simulink model "base_model_lqeH"  (R2020b)
settings: Solver=ode1  StartTime=0  StopTime=1150  FixedStep=0.1  RelTol=1e-3
libraries: simulink_extras x33
(part 1 of 3)
settings Model: Creator=LEON  LastModifiedBy=leonk
settings DataIOCC: ReturnWorkspaceOutputs=off
settings OptimizationCC: DefaultParameterBehavior=Inlined  EnhancedBackFolding=on  PassReuseOutputArgsAs=Individual arguments  ZeroExternalMemoryAtStartup=off  ZeroInternalMemoryAtStartup=off  OptimizeBlockOrder=speed  DifferentSizesBufferReuse=on  OptimizationCustomize=off  EfficientTunableParamExpr=on
settings DebuggingCC: ParameterTunabilityLossMsg=error  ArithmeticOperatorsInVariantConditions=warning
settings SFSimCC: MATLABDynamicMemAlloc=off  CustomCodeUndefinedFunction=UseInterfaceOnly
settings RTWCC: Description=Embedded Coder  SystemTargetFile=ert.tlc  GenCodeOnly=on  TemplateMakefile=ert_default_tmf
settings CodeAppCC: ForceParamTrailComments=on  IgnoreCustomStorageClasses=off  OperatorAnnotations=on  SimulinkDataObjDesc=on  SFDataObjDesc=on  InsertBlockDesc=on
settings ERTTargetCC: TargetLangStandard=C99 (ISO)  GenerateSampleERTMain=on  InlinedParameterPlacement=NonHierarchical  ERTCustomFileTemplate=example_file_process.tlc

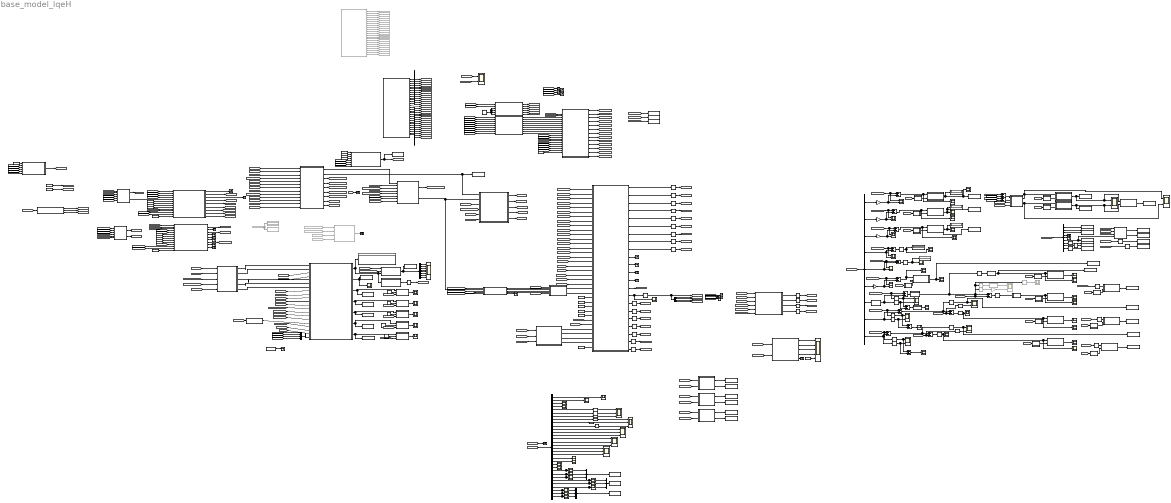
== system base_model_lqeH ==
  note: alpha&betta&gamma
  note: Ve&Vn
  note: lat&lon
  note: sat2Params
  note: sat3Params
  note: sat1Params
  note: time
  note: Altitude
  note: Алгориттм БИНС
  note: Егор
  note: Без базового спутника
  note: Корнтроль измерений
  note: Autoreloader
     {21..22,24,28..33,40..50} (20 alike) : Scope
     {23,26..27,34..35,37..39} (8 alike) : Scope  NumInputPorts=2
  "   25" : Scope  Commented=on  NumInputPorts=2
  "   36" : Scope  Commented=on
  "  3" : Scope
  " 12" : Scope
  " 13" : Scope
  " 14" : Scope  NumInputPorts=2
  " 15" : Scope  NumInputPorts=2
  " 16" : Scope  NumInputPorts=2
  ADD error SAT : MATLAB Function  TreatAsAtomicUnit=on
  Constant{,3..5,8..14,34,36} (13 alike) : Constant  Value=0
  Constant1 : Constant
  Constant{15,19..20,22} (4 alike) : Constant  OutDataTypeStr=uint8
  Constant16 : Constant  Value=[1, 1, 0.4, 10]
  Constant17 : Constant  Value=3
  Constant18 : Constant  Value=8  OutDataTypeStr=uint8
  Constant2 : Constant  Value=15
  Constant21 : Constant  Value=0  OutDataTypeStr=uint8
  Constant23 : Constant  Value=1000
  Constant28 : Constant  Value=8
  Constant29 : Constant  Value=50
  Constant30 : Constant  Value=0  OutDataTypeStr=uint8
  Constant31 : Constant  Value=500
  Constant32 : Constant  Value=800
  Constant33 : Constant  Value=1200
  Constant35 : Constant
  Constant6 : Constant  Value=10
  Constant7 : Constant  Value=10
  DOPS : MATLAB Function  TreatAsAtomicUnit=on
  Demux : Demux  Outputs=32
  Demux2 : Demux
  Demux4 : Demux  Outputs=8
  Demux5 : Demux  Outputs=9
  Demux6 : Demux  Outputs=9
  Display11 : Display  Commented=on
  Display{12,23,29..32} (6 alike) : Display
  FormZ : MATLAB Function  TreatAsAtomicUnit=on
  From168 : From  Commented=on  GotoTag=satVisible
  From270 : From  Commented=on  GotoTag=psdRange_GNSSvis
  From289 : From  Commented=on  GotoTag=satCoefs
  From291 : From  Commented=on  GotoTag=satIDvis
  From298 : From  Commented=on  GotoTag=satInctrl
  Fuck matlab1 : MATLAB Function  TreatAsAtomicUnit=on
  Fuck matlab10 : MATLAB Function  Commented=on  TreatAsAtomicUnit=on
  Fuck matlab11 : MATLAB Function  TreatAsAtomicUnit=on
  Fuck matlab2 : MATLAB Function  TreatAsAtomicUnit=on
  Fuck matlab3 : MATLAB Function  TreatAsAtomicUnit=on
  Fuck matlab4 : MATLAB Function  TreatAsAtomicUnit=on
  Fuck matlab5 : MATLAB Function  TreatAsAtomicUnit=on
  Fuck matlab6 : MATLAB Function  TreatAsAtomicUnit=on
  Fuck matlab7 : MATLAB Function  TreatAsAtomicUnit=on
  Fuck matlab8 : MATLAB Function  TreatAsAtomicUnit=on
  Fuck matlab9 : MATLAB Function  TreatAsAtomicUnit=on
  GNNS_freq_imitetor : MATLAB Function  TreatAsAtomicUnit=on
  GNNS_freq_imitetor1 : MATLAB Function  TreatAsAtomicUnit=on
  GNSS_integrity_control1 : MATLAB Function  TreatAsAtomicUnit=on
  GNSS_receiver_imitator10 : MATLAB Function  TreatAsAtomicUnit=on
  GNSS_receiver_imitator6 : MATLAB Function  TreatAsAtomicUnit=on
  GNSS_receiver_imitator7 : MATLAB Function  TreatAsAtomicUnit=on
  GNSS_receiver_imitator8 : MATLAB Function  TreatAsAtomicUnit=on
  GNSS_receiver_imitator9 : MATLAB Function  TreatAsAtomicUnit=on
  GSK->DGSK : MATLAB Function  TreatAsAtomicUnit=on
  GSK->DGSK1 : MATLAB Function  TreatAsAtomicUnit=on
  Goto1 : Goto  Commented=on  GotoTag=ACC_data
  Goto10 : Goto  Commented=on  GotoTag=ic_Vh
  Goto11 : Goto  Commented=on  GotoTag=time_shift
  Goto112 : Goto  Commented=on  GotoTag=satStartTime
  Goto12 : Goto  Commented=on  GotoTag=GRS_data
  Goto129 : Goto  Commented=on  GotoTag=offSet_Vn
  Goto136 : Goto  Commented=on  GotoTag=satStopTime
  Goto137 : Goto  Commented=on  GotoTag=offSet_Ve
  Goto138 : Goto  Commented=on  GotoTag=offSet_Vh
  Goto139 : Goto  Commented=on  GotoTag=offSet_lat
  Goto140 : Goto  Commented=on  GotoTag=offSet_lon
  Goto141 : Goto  Commented=on  GotoTag=offSet_alt
  Goto145 : Goto  Commented=on  GotoTag=satDeltaUp
  Goto146 : Goto  Commented=on  GotoTag=satDeltaDown
  Goto2 : Goto  Commented=on  GotoTag=ic_heading
  Goto3 : Goto  Commented=on  GotoTag=ic_pitch
  Goto4 : Goto  Commented=on  GotoTag=ic_roll
  Goto48 : Goto  Commented=on  GotoTag=ctrl_data
  Goto5 : Goto  Commented=on  GotoTag=ic_lat
  Goto6 : Goto  Commented=on  GotoTag=ic_lon
  Goto7 : Goto  Commented=on  GotoTag=ic_Ve
  Goto8 : Goto  Commented=on  GotoTag=ic_Vn
  Goto9 : Goto  Commented=on  GotoTag=ic_alt
  INS mesurment model : MATLAB Function  TreatAsAtomicUnit=on
  MATLAB Function3 : MATLAB Function  Commented=on  TreatAsAtomicUnit=on
  MATLAB Function4 : MATLAB Function  TreatAsAtomicUnit=on
  Memory{1,16..27,29..37} (22 alike) : Memory
  Model : ModelReference  ModelNameDialog=SINS_model_3ch_h.slx  SimulationMode=Normal  ModelReferenceVersion=5.358
  Model2 : ModelReference  ModelNameDialog=lqe_ins_h.slx  SimulationMode=Normal  ModelReferenceVersion=5.1159
  Mux : Mux  Inputs=3
  Mux1 : Mux  Inputs=3
  Mux2 : Mux  Inputs=3
  Mux3 : Mux
  Pitch_1 : simulink_extras/Transformations/Radians to Degrees
  Pitch_err   1 : simulink_extras/Transformations/Radians to Degrees
  Radians to Degrees{,13..14,17..19,22,27..29,31} (11 alike) : simulink_extras/Transformations/Radians to Degrees
  Radians to Degrees21 : simulink_extras/Transformations/Radians to Degrees  Commented=on
  Roll_err   1 : simulink_extras/Transformations/Radians to Degrees
  Scope{1..2,5..7,10..11,13..14,20..22,24..25,66,76..84} (24 alike) : Scope
  Scope{19,32,56..58} (5 alike) : Scope  NumInputPorts=3
  Scope3 : Scope  NumInputPorts=2
  Scope64 : Scope  NumInputPorts=8
  Scope8 : Scope  NumInputPorts=2
  Scope87 : Scope  NumInputPorts=5
  Scope9 : Scope  NumInputPorts=2
  StaPosition : MATLAB Function  TreatAsAtomicUnit=on
  Terminator{,1..27} (28 alike) : Terminator
  To Workspace1 : ToWorkspace  Commented=on  VariableName=satVisibleCount  SampleTime=-1
  To Workspace10 : ToWorkspace  VariableName=satIC_2cfs  SampleTime=-1
  To Workspace11 : ToWorkspace  VariableName=satIC_3cfs  SampleTime=-1
  To Workspace12 : ToWorkspace  VariableName=satIC_3ID  SampleTime=-1
  To Workspace13 : ToWorkspace  VariableName=satIC_1P  SampleTime=-1
  To Workspace14 : ToWorkspace  VariableName=satIC_2P  SampleTime=-1
  To Workspace15 : ToWorkspace  VariableName=d_heading  SampleTime=-1
  To Workspace16 : ToWorkspace  VariableName=satIC_3P  SampleTime=-1
  To Workspace17 : ToWorkspace  VariableName=pitch_err  SampleTime=-1
  To Workspace18 : ToWorkspace  VariableName=roll_err  SampleTime=-1
  To Workspace19 : ToWorkspace  VariableName=d_roll  SampleTime=-1
  To Workspace2 : ToWorkspace  VariableName=slowZLevel  SampleTime=-1
  To Workspace20 : ToWorkspace  VariableName=Ve_REF  SampleTime=-1
  To Workspace21 : ToWorkspace  VariableName=Vn_REF  SampleTime=-1
  To Workspace22 : ToWorkspace  VariableName=Vh_REF  SampleTime=-1
  To Workspace23 : ToWorkspace  VariableName=Y_REF  SampleTime=-1
  To Workspace24 : ToWorkspace  VariableName=X_REF  SampleTime=-1
  To Workspace25 : ToWorkspace  VariableName=alt_REF  SampleTime=-1
  To Workspace26 : ToWorkspace  VariableName=heading_REF  SampleTime=-1
  To Workspace27 : ToWorkspace  VariableName=pitch_REF  SampleTime=-1
  To Workspace28 : ToWorkspace  VariableName=roll_REF  SampleTime=-1
  To Workspace29 : ToWorkspace  VariableName=lat_REF  SampleTime=-1
  To Workspace3 : ToWorkspace  VariableName=latSINS  SampleTime=-1
  To Workspace30 : ToWorkspace  VariableName=lon_REF  SampleTime=-1
  To Workspace31 : ToWorkspace  VariableName=Ve_err  SampleTime=-1
  To Workspace32 : ToWorkspace  VariableName=Vn_err  SampleTime=-1
  To Workspace33 : ToWorkspace  VariableName=Vh_err  SampleTime=-1
  To Workspace34 : ToWorkspace  VariableName=lat_err  SampleTime=-1
  To Workspace35 : ToWorkspace  VariableName=lon_err  SampleTime=-1
  To Workspace36 : ToWorkspace  VariableName=alt_err  SampleTime=-1
  To Workspace37 : ToWorkspace  VariableName=heading_err  SampleTime=-1
  To Workspace38 : ToWorkspace  VariableName=intCtrl_status  SampleTime=-1
  To Workspace39 : ToWorkspace  VariableName=fastCriteriaLevel  SampleTime=-1
  To Workspace4 : ToWorkspace  VariableName=psdErr  SampleTime=-1
  To Workspace40 : ToWorkspace  VariableName=slowMeanLevel  SampleTime=-1
  To Workspace41 : ToWorkspace  VariableName=fastLevel  SampleTime=-1
  To Workspace42 : ToWorkspace  VariableName=lonSINS  SampleTime=-1
  To Workspace43 : ToWorkspace  VariableName=altSINS  SampleTime=-1
  To Workspace44 : ToWorkspace  VariableName=slowZCriteria  SampleTime=-1
  To Workspace45 : ToWorkspace  VariableName=satVisibleCount  SampleTime=-1
  To Workspace46 : ToWorkspace  VariableName=crdErr  SampleTime=-1
  To Workspace5 : ToWorkspace  VariableName=satAV  SampleTime=-1
  To Workspace6 : ToWorkspace  VariableName=d_pitch  SampleTime=-1
  To Workspace7 : ToWorkspace  VariableName=satIC_1ID  SampleTime=-1
  To Workspace8 : ToWorkspace  VariableName=satIC_1cfs  SampleTime=-1
  To Workspace9 : ToWorkspace  VariableName=satIC_2ID  SampleTime=-1
  "Ve_err   " : Sum  Inputs=+-
  Ve_err 1 : MATLAB Function  TreatAsAtomicUnit=on
  "Vh_err  " : Sum  Inputs=+-
  Vh_err 1 : MATLAB Function  TreatAsAtomicUnit=on
  "Vn_err  " : Sum  Inputs=+-
  Vn_err 1 : MATLAB Function  TreatAsAtomicUnit=on
  "alt_err    " : Sum  Inputs=+-
  alt_err 1 : MATLAB Function  TreatAsAtomicUnit=on
  altimetrImitator : MATLAB Function  TreatAsAtomicUnit=on
  altimetrImitator1 : MATLAB Function  TreatAsAtomicUnit=on
  bigHeadingFix1 : MATLAB Function  TreatAsAtomicUnit=on
  bigHeadingFix2 : MATLAB Function  TreatAsAtomicUnit=on
  coord_err7 : MATLAB Function  TreatAsAtomicUnit=on
  coord_err8 : MATLAB Function  TreatAsAtomicUnit=on
  crtl_Ve1 : Gain
  crtl_Vh1 : Gain
  crtl_Vn1 : Gain
  crtl_altitude1 : Gain
  d_heading1 : Gain  Commented=on
  d_pitch1 : simulink_extras/Transformations/Radians to Degrees
  d_roll1 : simulink_extras/Transformations/Radians to Degrees
  heading_3 : simulink_extras/Transformations/Radians to Degrees
  heading_4 : simulink_extras/Transformations/Radians to Degrees  Commented=on
  heading_5 : simulink_extras/Transformations/Radians to Degrees  Commented=on
  heading_6 : simulink_extras/Transformations/Radians to Degrees
  heading_INS  1 : MATLAB Function  Commented=on  TreatAsAtomicUnit=on
  heading_INS  2 : MATLAB Function  TreatAsAtomicUnit=on
  "heading_err     " : MATLAB Function  TreatAsAtomicUnit=on
  heading_err     1 : MATLAB Function  TreatAsAtomicUnit=on
  heading_err     2 : MATLAB Function  TreatAsAtomicUnit=on
  heading_err     3 : MATLAB Function  TreatAsAtomicUnit=on
  heading_err     4 : MATLAB Function  TreatAsAtomicUnit=on
  heading_err    {1..9} (9 alike) : simulink_extras/Transformations/Radians to Degrees
  heading_err  1 : MATLAB Function  TreatAsAtomicUnit=on
  heading_err1 : Sum  Inputs=+-
  heading_err_FBon 2 : MATLAB Function  TreatAsAtomicUnit=on
  heading_err_FBon1 : Sum  Inputs=+-
  lat_err 1 : MATLAB Function  TreatAsAtomicUnit=on
  lat_err 2 : MATLAB Function  TreatAsAtomicUnit=on
  lat_err3 : Sum  Inputs=+-
  lat_err4 : Sum  Inputs=+-
  lon_err 1 : MATLAB Function  TreatAsAtomicUnit=on
  lon_err3 : Sum  Inputs=+-
  lon_err4 : Sum  Inputs=+-
  lqe_coord_cor2 : MATLAB Function  TreatAsAtomicUnit=on
  "pitch_err    " : MATLAB Function  TreatAsAtomicUnit=on
  pitch_err 1 : simulink_extras/Transformations/Radians to Degrees
  pitch_err1 : Sum  Inputs=+-
  pitch_err_FBon1 : Sum  Inputs=+-
  psdRange_Sat : ModelReference  ModelNameDialog=psdRange_model.slx  SimulationMode=Normal  ModelReferenceVersion=1.113
      settings: PortSchema="{\"entries\":[{\"content\":{\"sides\":[{\"content\":{\"connectorIds\":[\"In1\",\"In2\",\"In3\",\"In4\",\"In5\",\"In6\",\"In8\",\"In7\",\"In9\",\"In10\",\"In11\",\"In12\",\"In13\",\"In14\"]},\"type\":\"ConnectorPlacement.EquallySpacedRectSide\",\"uuid\":\"0992fbca-6c1d-43ca-af68-52a1663360d0\"},{\"content\":{\"connectorIds\":[\"Out1\",\"Out2\",\"Out3\",\"Out4\",\"Out5\",\"Out6\",\"Out7\",\"Out8\",\"Out9\"],\"side\":\"RIGHT\"},\"type\":\"ConnectorPlacement.EquallySpacedRectSide\",\"uuid\":\"279fbf8e-dc69-40a1-ad66-d0ae37456352\"},{\"content\":{\"connectorIds\":[],\"side\":\"TOP\"},\"type\":\"ConnectorPlacement.EquallySpacedRectSide\",\"uuid\":\"4e5886c2-56d5-49fe-96a3-fea858babac4\"},{\"content\":{\"connectorIds\":[],\"side\":\"HIDDEN\"},\"type\":\"ConnectorPlacement.EquallySpacedRectSide\",\"uuid\":\"b5bcda28-ff0f-4448-99fe-4545b2b7e269\"}]},\"type\":\"ConnectorPlacement.EquallySpacedConnector\",\"uuid\":\"877d5e3f-f6cf-4aa5-86c3-e38699d2b886\"}],\"packageUris\":[\"http://schema.mathworks.com/mf0/Connector/R2020b\"],\"version\":\"1.0\"}"
  psdRange_Sat1 : ModelReference  ModelNameDialog=psdRange_model.slx  SimulationMode=Normal  ModelReferenceVersion=1.113
      settings: PortSchema="{\"entries\":[{\"content\":{\"sides\":[{\"content\":{\"connectorIds\":[\"In1\",\"In2\",\"In3\",\"In4\",\"In5\",\"In6\",\"In8\",\"In7\",\"In9\",\"In10\",\"In11\",\"In12\",\"In13\",\"In14\"]},\"type\":\"ConnectorPlacement.EquallySpacedRectSide\",\"uuid\":\"0992fbca-6c1d-43ca-af68-52a1663360d0\"},{\"content\":{\"connectorIds\":[\"Out1\",\"Out2\",\"Out3\",\"Out4\",\"Out5\",\"Out6\",\"Out7\",\"Out8\",\"Out9\"],\"side\":\"RIGHT\"},\"type\":\"ConnectorPlacement.EquallySpacedRectSide\",\"uuid\":\"279fbf8e-dc69-40a1-ad66-d0ae37456352\"},{\"content\":{\"connectorIds\":[],\"side\":\"TOP\"},\"type\":\"ConnectorPlacement.EquallySpacedRectSide\",\"uuid\":\"4e5886c2-56d5-49fe-96a3-fea858babac4\"},{\"content\":{\"connectorIds\":[],\"side\":\"HIDDEN\"},\"type\":\"ConnectorPlacement.EquallySpacedRectSide\",\"uuid\":\"b5bcda28-ff0f-4448-99fe-4545b2b7e269\"}]},\"type\":\"ConnectorPlacement.EquallySpacedConnector\",\"uuid\":\"877d5e3f-f6cf-4aa5-86c3-e38699d2b886\"}],\"packageUris\":[\"http://schema.mathworks.com/mf0/Connector/R2020b\"],\"version\":\"1.0\"}"
  roll_1 : simulink_extras/Transformations/Radians to Degrees
  "roll_err     " : MATLAB Function  TreatAsAtomicUnit=on
  roll_err 1 : simulink_extras/Transformations/Radians to Degrees
  roll_err{4..7} (4 alike) : Sum  Inputs=+-
  roll_err_FBon1 : Sum  Inputs=+-
  seter1 : MATLAB Function  TreatAsAtomicUnit=on
  seter10 : MATLAB Function  TreatAsAtomicUnit=on
  seter11 : MATLAB Function  TreatAsAtomicUnit=on
  seter12 : MATLAB Function  TreatAsAtomicUnit=on
  seter13 : MATLAB Function  TreatAsAtomicUnit=on
  seter2 : MATLAB Function  TreatAsAtomicUnit=on
  seter3 : MATLAB Function  TreatAsAtomicUnit=on
  seter4 : MATLAB Function  TreatAsAtomicUnit=on
  seter5 : MATLAB Function  TreatAsAtomicUnit=on
  seter6 : MATLAB Function  TreatAsAtomicUnit=on
  seter7 : MATLAB Function  TreatAsAtomicUnit=on
  seter8 : MATLAB Function  TreatAsAtomicUnit=on
  seter9 : MATLAB Function  TreatAsAtomicUnit=on
  wires:
  MATLAB Function3/1(GRS) -> Goto12/1
  MATLAB Function3/2(ACC) -> Goto1/1
  MATLAB Function3/3(heading) -> Goto2/1
  MATLAB Function3/4(pitch) -> Goto3/1
  MATLAB Function3/5(roll) -> Goto4/1
  MATLAB Function3/7(lon) -> Goto6/1
  MATLAB Function3/6(lat) -> Goto5/1
  MATLAB Function3/8(Ve) -> Goto7/1
  MATLAB Function3/9(Vn) -> Goto8/1
  MATLAB Function3/12(time_shft) -> Goto11/1
  MATLAB Function3/11(Vh) -> Goto10/1
  MATLAB Function3/10(H) -> Goto9/1
  Model/1 -> [SINS_Ve]
  Model/2 -> [SINS_Vn]
  Model/4 -> [SINS_latitude]
  Model/3 -> [SINS_Vh]
  Model/5 -> [SINS_longitude]
  Demux/14 -> Scope32/1
  Demux/4 -> Scope24/1
  Radians to Degrees13/1 -> Scope19/2
  Demux/15 -> Scope32/2
  Demux/7 -> Radians to Degrees14/1
  Radians to Degrees/1 -> Scope19/1
  Demux/16 -> Scope32/3
  Demux/5 -> Radians to Degrees/1
  Demux/6 -> Radians to Degrees13/1
  Demux/1 -> Scope20/1
  Demux/3 -> Scope22/1
  Radians to Degrees14/1 -> Scope19/3
  Demux/2 -> Scope21/1
  [GRS_data] -> INS mesurment model/1(grs_ideal)
  [ACC_data] -> INS mesurment model/2(acc_ideal)
  [ic_roll] -> lqe_coord_cor2/3(roll)
  [ic_pitch] -> lqe_coord_cor2/2(pitch)
  [ic_heading] -> lqe_coord_cor2/1(heading)
  [ic_Vn] -> lqe_coord_cor2/8(Vn)
  [ic_Ve] -> lqe_coord_cor2/7(Ve)
  [ic_lat] -> lqe_coord_cor2/4(lat)
  [ic_lon] -> lqe_coord_cor2/5(lon)
  Demux/8 -> Radians to Degrees17/1
  Demux/9 -> Radians to Degrees18/1
  Demux/10 -> Radians to Degrees19/1
  Demux/17 -> Scope58/1
  Demux/18 -> Scope58/2
  Demux/19 -> Scope58/3
  Radians to Degrees17/1 -> Scope56/1
  Demux/12 -> Scope57/2
  Demux/13 -> Scope57/3
  Demux/11 -> Scope57/1
  Radians to Degrees18/1 -> Scope56/2
  Radians to Degrees19/1 -> Scope56/3
  INS mesurment model/1(grs_data) -> [GRS_real]
  INS mesurment model/2(acc_data) -> [ACC_real]
  Model/7 -> [SINS_heading]
  Model/8 -> [SINS_pitch]
  Model/9 -> [SINS_roll]
  Model/10 -> [SINS_nGSK]
  Model/11 -> [SINS_OmgGSK]
  Model/12 -> [SINS_matDirCos]
  Model/6 -> [SINS_altitude]
  [amnd_matDirCos] -> Model/13
  Constant12/1 -> Model/21
  [ic_Vh] -> lqe_coord_cor2/9(Vh)
  [ic_alt] -> lqe_coord_cor2/6(alt)
  Demux/20 -> Scope76/1
  Demux/21 -> Scope5/1
  [time_shift] -> Model/20
  [lqe_dVn] -> Model/18
  [lqe_dVe] -> Model/17
  [lqe_dlon] -> Model/15
  [lqe_dlat] -> Model/14
  [lqe_dalt] -> Model/16
  [lqe_dVh] -> Model/19
  [lqe_ctrl] -> Model/12
  lqe_coord_cor2/9(Vh_0) -> Model/11
  lqe_coord_cor2/8(Vn_0) -> Model/10
  lqe_coord_cor2/7(Ve_0) -> Model/9
  lqe_coord_cor2/6(alt_0) -> Model/8
  lqe_coord_cor2/5(lon_0) -> Model/7
  lqe_coord_cor2/1(heading_0) -> Model/3
  lqe_coord_cor2/2(pitch_0) -> Model/4
  lqe_coord_cor2/3(roll_0) -> Model/5
  lqe_coord_cor2/4(lat_0) -> Model/6
  MATLAB Function3/13(cntrl_data) -> Goto48/1
  [ACC_real] -> Model/2
  [GRS_real] -> Model/1
  Model/13 -> [SINS_dVGSK]
  INS mesurment model/6(dK_grs) -> [dKgrs]
  Constant/1 -> INS mesurment model/4(n2), INS mesurment model/3(n1), INS mesurment model/5(n3), INS mesurment model/6(n4)
  INS mesurment model/3(dacc) -> [dacc]
  INS mesurment model/4(dgrs) -> [dgrs]
  INS mesurment model/5(dK_acc) -> [dKacc]
  [time_shift] -> StaPosition/1(time_shift)
  StaPosition/1(satCounter) -> [satCount]
  StaPosition/2(satPosVel) -> [satPosVel]
  Constant2/1 -> [elevMask]
  psdRange_Sat/1 -> Terminator/1
  psdRange_Sat/2 -> [psdRange_sat]
  psdRange_Sat/3 -> Terminator1/1
  psdRange_Sat/4 -> [psdVel_sat]
  StaPosition/3(satHealth) -> [satHealth]
  psdRange_Sat/5 -> [dPsdRange]
  [satVisible] -> FormZ/1(satVisible)
  [satCount] -> FormZ/2(satCount)
  psdRange_Sat/6 -> [satVisible]
  [satVisibleFlag_GNSS] -> FormZ/4(satVisibleFlag_GNSS)
  psdRange_Sat1/2 -> Terminator2/1
  psdRange_Sat1/4 -> Terminator3/1
  psdRange_Sat1/3 -> [psdVel_INS]
  psdRange_Sat1/1 -> [psdRange_INS]
  [psdVel_INS] -> FormZ/7(psdVel_INS)
  [psdRange_INS] -> FormZ/6(psdRange_INS)
  [psdRange_sat] -> FormZ/5(psdRange_sat)
  [psdVel_sat] -> FormZ/8(psdVel_sat)
  [time_shift] -> GNNS_freq_imitetor/3(time_shift)
  GNNS_freq_imitetor/1(satInfo) -> [satInfo_shrt]
  GNNS_freq_imitetor/3(timeDelay) -> [timeDelayGNSS]
  GNNS_freq_imitetor/4(frameAvalible_GNSS) -> [frameAvalible]
  psdRange_Sat1/5 -> Terminator4/1
  psdRange_Sat1/6 -> Terminator5/1
  FormZ/2(satNum) -> To Workspace45/1, GNNS_freq_imitetor/1(satNum_AV)
  GSK->DGSK1/1(pos) -> [posObjINS]
  GSK->DGSK1/2(vel) -> [velObjINS]
  FormZ/3(psdRange_INS_short) -> [psdRange_INSvis]
  FormZ/1(satInfo) -> ADD error SAT/1(satInfo)
  [GRS_real] -> Model2/11
  [SINS_dVGSK] -> Model2/15
  [ACC_real] -> Model2/13
  [SINS_nGSK] -> Model2/14
  [SINS_latitude] -> Model2/1
  [SINS_altitude] -> Model2/3
  [SINS_Vh] -> Model2/6
  [SINS_OmgGSK] -> Model2/12
  [SINS_roll] -> Model2/9
  [SINS_Vn] -> Model2/5
  [SINS_longitude] -> Model2/2
  [SINS_Ve] -> Model2/4
  [SINS_pitch] -> Model2/8
  [time_shift] -> Model2/16
  [SINS_matDirCos] -> Model2/10
  [SINS_heading] -> Model2/7
  Constant18/1 -> [satCountPreset]
  [satPosVel] -> psdRange_Sat/2
  [satHealth] -> psdRange_Sat/3
  [satCount] -> psdRange_Sat/1
  GSK->DGSK/2(vel) -> psdRange_Sat/5
  Constant8/1 -> psdRange_Sat/6
  Constant4/1 -> psdRange_Sat/7
  Constant5/1 -> psdRange_Sat/8
  Constant3/1 -> psdRange_Sat/9
  Constant1/1 -> GNNS_freq_imitetor1/1(dispSat)
  [elevMask] -> psdRange_Sat/11
  [satPosVel] -> psdRange_Sat1/2
  [satCount] -> psdRange_Sat1/1
  [satHealth] -> psdRange_Sat1/3
  [posObjINS] -> psdRange_Sat1/4
  [velObjINS] -> psdRange_Sat1/5
  Constant14/1 -> psdRange_Sat1/6
  Constant13/1 -> psdRange_Sat1/8
  Constant11/1 -> psdRange_Sat1/7
  Constant10/1 -> psdRange_Sat1/9
  Constant9/1 -> psdRange_Sat1/10
  [elevMask] -> psdRange_Sat1/11
  [satCountPreset] -> FormZ/3(satCountPreset)
  [satVisibleFlag_INS] -> FormZ/9(satVisibleFlag_INS)
  FormZ/5(satPosVel_short) -> [satPosVel_short]
  [satPosVel_short] -> GNNS_freq_imitetor/4(satPosVel_AV)
  GNNS_freq_imitetor/5(satPosVel) -> [satPosVel_shrt]
  [satPosVel] -> FormZ/10(satPosVel)
  [satPosVel_shrt] -> Model2/19
  [satInfo_shrt] -> Model2/18
  [frameAvalible] -> Model2/20
  GNNS_freq_imitetor/2(satNum) -> [satNumInZ]
  [satNumInZ] -> Model2/21
  [timeDelayGNSS] -> Model2/17
  From168/1 -> Display11/1, To Workspace1/1
  [satCountPreset] -> Model2/22
  Constant23/1 -> Model2/25
  Constant19/1 -> Model2/26
  Constant20/1 -> Model2/27
  Constant21/1 -> Model2/28
  Constant22/1 -> Model2/29
  Demux/23 -> Scope25/1
  Demux/22 -> Scope6/1
  Memory29/1 -> [alpha2]
  Memory26/1 -> Demux2/1, [lqe_ctrl]
  GNSS_receiver_imitator6/4(matr_CORR) -> Memory23/1
  Memory21/1 -> [d_roll]
  Memory22/1 -> [d_pitch]
  GNSS_receiver_imitator6/3(droll) -> Memory21/1
  GNSS_receiver_imitator6/2(dpitch) -> Memory22/1
  Memory30/1 -> [gamma2]
  [beta2] -> GNSS_receiver_imitator6/2(beta)
  [gamma2] -> GNSS_receiver_imitator6/3(gamma)
  Memory25/1 -> [lqe_dVh]
  Memory17/1 -> [lqe_dlon]
  [SINS_heading] -> GNSS_receiver_imitator6/4(heading)
  [alpha2] -> GNSS_receiver_imitator6/1(alpha)
  Model2/15 -> Scope7/1, Memory26/1
  Memory24/1 -> [lqe_dVe]
  Memory19/1 -> [lqe_dVn]
  Memory18/1 -> [beta2]
  [SINS_pitch] -> GNSS_receiver_imitator6/5(pitch)
  Memory23/1 -> [amnd_matDirCos]
  [SINS_roll] -> GNSS_receiver_imitator6/6(roll)
  Memory16/1 -> [lqe_dlat]
  Memory27/1 -> [d_yaw]
  Memory20/1 -> [lqe_dalt]
  GNSS_receiver_imitator6/1(dyaw) -> Memory27/1
  Model2/14 -> [lqe_P]
  [lqe_P] -> Demux/1
  Model2/1 -> Memory16/1
  Model2/2 -> Memory17/1
  Model2/3 -> Memory20/1
  Model2/4 -> Memory24/1
  Model2/5 -> Memory19/1
  Model2/6 -> Memory25/1
  Model2/7 -> Memory29/1
  Model2/8 -> Memory18/1
  Model2/9 -> Memory30/1
  psdRange_Sat/7 -> [satVisibleFlag_GNSS]
  [dPsdRange] -> FormZ/11(dPsdRange)
  FormZ/6(sigmPsdRange) -> [sigmPrdRange]
  psdRange_Sat1/7 -> [satVisibleFlag_INS]
  altimetrImitator1/2(sigmPsdVel) -> Model2/24
  [satPosVel_short] -> DOPS/1(satPosVel)
  [satVisible] -> DOPS/4(satCountPreset)
  Demux2/1 -> [ctrl_pos]
  Demux2/4 -> [ctrl_alt]
  Demux2/3 -> [ctrl_ang]
  Demux2/2 -> [ctrl_vel]
  FormZ/7(satIDvis) -> [satIDvis]
  [psdRange_SATvis] -> DOPS/3(psdRange_GNSS_short)
  psdRange_Sat1/8 -> Terminator6/1
  psdRange_Sat1/9 -> Terminator7/1
  psdRange_Sat/9 -> [satElevation]
  psdRange_Sat/8 -> [satAzimut]
  [satElevation] -> FormZ/13(satElevation)
  [satAzimut] -> FormZ/12(satAzimut)
  FormZ/8(satAzimutVis) -> [satAzimutVis]
  FormZ/9(satEleavtionVis) -> [satElevationVis]
  Model2/17 -> Memory32/1
  Model2/16 -> Memory31/1
  Model2/18 -> Memory33/1
  Model2/19 -> Memory34/1
  [DispSat] -> psdRange_Sat/10
  FormZ/4(psdRange_GNSS_short) -> [psdRange_SATvis]
  Demux4/6 -> Scope64/6
  Demux4/5 -> Scope64/5
  GNSS_integrity_control1/5(slowCritLevel) -> Fuck matlab3/1(data), To Workspace40/1
  [satIDvis] -> Fuck matlab6/2(satID_shrt)
  Demux4/8 -> Scope64/8
  Fuck matlab6/1(satAv) -> Demux4/1, To Workspace5/1
  Demux4/2 -> Scope64/2
  [DispSat] -> Fuck matlab7/1(size)
  [satCountPreset] -> Fuck matlab5/5(satCountPreset)
  [satPosVel_short] -> GNSS_integrity_control1/13(satPosVel)
  [LQE_L] -> GNSS_integrity_control1/10(lqe_L)
  Fuck matlab5/4(psdRange_GNSSvis_fix) -> GNSS_integrity_control1/6(psdRangeGNSS_in)
  GNSS_integrity_control1/1(satID_IC) -> Fuck matlab9/1(satID_IC), Fuck matlab6/3(satID_IC), Display23/1
  Fuck matlab5/3(psdRange_INSvis_fix) -> GNSS_integrity_control1/5(psdRangeINS_in)
  [satIDvis] -> Fuck matlab5/2(satIDs)
  Fuck matlab5/2(satIDs_fix) -> GNSS_integrity_control1/2(satID_in)
  [satVisible] -> Fuck matlab5/1(satVisible)
  [SINS_longitude] -> GNSS_integrity_control1/15(lon)
  [LQE_F] -> GNSS_integrity_control1/8(lqe_F)
  [psdRange_INSvis] -> Fuck matlab5/3(psdRange_INSvis)
  [satVisible] -> Fuck matlab6/1(satVisible)
  [LQE_P] -> GNSS_integrity_control1/9(lqe_P)
  [SINS_latitude] -> GNSS_integrity_control1/14(lat)
  [SINS_altitude] -> GNSS_integrity_control1/16(alt)
  Demux4/3 -> Scope64/3
  [LQE_Q] -> GNSS_integrity_control1/11(lqe_Q)
  [satElevationVis] -> GNSS_integrity_control1/4(satElevation_in)
  GNSS_integrity_control1/2(intCtrl_status) -> Scope66/1, To Workspace38/1
  Demux4/7 -> Scope64/7
  Fuck matlab7/1(psdRMiss) -> GNSS_integrity_control1/17(disp_SatPos)
  Fuck matlab5/5(baseSatID) -> GNSS_integrity_control1/7(baseSatID)
  [frameAvalible] -> GNSS_integrity_control1/18(frameAvalible)
  Demux4/4 -> Scope64/4
  [posObjINS] -> GNSS_integrity_control1/12(posObjINS)
  Fuck matlab5/1(satNum) -> GNSS_integrity_control1/1(satNum)
  Demux4/1 -> Scope64/1
  [satAzimutVis] -> GNSS_integrity_control1/3(satAzimut_in)
  Fuck matlab9/1(satID_forCtrl) -> Memory36/1
  Demux/25 -> Mux/2, Scope77/1
  Demux/26 -> Mux/3, Scope78/1
  Memory31/1 -> [LQE_F]
  Memory32/1 -> [LQE_P]
  Memory33/1 -> [LQE_L]
  Memory34/1 -> [LQE_Q]
  [satIDvis] -> Model2/31
  Model2/20 -> Memory35/1
  Memory35/1 -> [satCoefs]
  [sat_intCtrl] -> Model2/30
  [psdRangeSat_spuf] -> Fuck matlab5/4(psdRange_GNSSvis)
  Memory36/1 -> [sat_intCtrl]
  [ic_alt] -> altimetrImitator/1(alt_ideal)
  [ic_Vh] -> altimetrImitator/2(Vh)
  [time_shift] -> altimetrImitator/3(time_shift)
  altimetrImitator/4(timeStep) -> Model2/35
  altimetrImitator/3(isAltAvalible) -> Model2/34
  altimetrImitator/1(Alt) -> Model2/32
  [satCoefs] -> GNSS_receiver_imitator7/1(satCoefs)
  GNSS_receiver_imitator7/1(sat1_id) -> Scope87/1
  GNSS_receiver_imitator7/2(sat1_a) -> Scope87/2
  GNSS_receiver_imitator7/3(sat1_b) -> Scope87/3
  GNSS_receiver_imitator7/4(sat1_c) -> Scope87/4
  GNSS_receiver_imitator7/5(sat1_t) -> Terminator25/1
  Memory37/1 -> [satInctrl]
  Model2/21 -> Memory37/1
  [satInctrl] -> GNSS_receiver_imitator7/2(satInctrl)
  altimetrImitator/2(RMS) -> Model2/33
  Constant31/1 -> Fuck matlab8/1(tStart)
  Constant32/1 -> Fuck matlab8/2(tp)
  Constant33/1 -> Fuck matlab8/3(tEnd)
  [satCoefs] -> GNSS_receiver_imitator8/1(satCoefs)
  [satInctrl] -> GNSS_receiver_imitator8/2(satInctrl)
  GNSS_receiver_imitator8/1(sat1_id) -> To Workspace7/1
  GNSS_receiver_imitator8/2(sat1_cfs) -> To Workspace8/1
  [satInctrl] -> GNSS_receiver_imitator9/2(satInctrl)
  [satCoefs] -> GNSS_receiver_imitator9/1(satCoefs)
  GNSS_receiver_imitator9/2(sat1_cfs) -> To Workspace10/1
  GNSS_receiver_imitator9/1(sat1_id) -> To Workspace9/1
  [satCoefs] -> GNSS_receiver_imitator10/1(satCoefs)
  GNSS_receiver_imitator10/2(sat1_cfs) -> To Workspace11/1
  GNSS_receiver_imitator10/1(sat1_id) -> To Workspace12/1
  [satInctrl] -> GNSS_receiver_imitator10/2(satInctrl)
  Mux/1 -> To Workspace13/1
  Demux/29 -> Mux1/3, Scope81/1
  Demux/27 -> Mux1/1, Scope79/1
  Mux1/1 -> To Workspace14/1
  Demux/28 -> Mux1/2, Scope80/1
  Demux/31 -> Mux2/2, Scope83/1
  Demux/30 -> Mux2/1, Scope84/1
  Demux/32 -> Mux2/3, Scope82/1
  Mux2/1 -> To Workspace16/1
  altimetrImitator1/1(sigmPsdRange) -> Model2/23
  [time_shift] -> altimetrImitator1/6(timeStep)
  DOPS/4(TDOP) -> altimetrImitator1/5(TDOP)
  DOPS/3(VDOP) -> altimetrImitator1/4(VDOP)
  DOPS/2(HDOP) -> altimetrImitator1/3(HDOP)
  DOPS/1(PDOP) -> altimetrImitator1/2(PDOP)
  coord_err7/2(y) -> Scope9/2, lon_err 1/1(data_in)
  [SINS_Vh] -> "   23"/1, "Vh_err  "/1
  [SINS_roll] -> roll_1/1, roll_err4/1
  heading_6/1 -> heading_INS  2/1(headingError)
  Demux5/3 -> crtl_Vh1/1
  heading_err    5/1 -> To Workspace30/1
  [SINS_pitch] -> pitch_err1/1, Pitch_1/1
  [d_roll] -> d_roll1/1, roll_err5/2
  Ve_err 1/1(data_out) -> To Workspace31/1, "   50"/1, Display12/1
  [ic_lat] -> lat_err4/2
  crtl_Ve1/1 -> "Ve_err   "/2, "   34"/2
  roll_err_FBon1/1 -> "   49"/1
  [d_yaw] -> Radians to Degrees21/1, roll_err7/2
  [SINS_Ve] -> "Ve_err   "/1, "   34"/1
  pitch_err_FBon1/1 -> " 12"/1
  heading_err_FBon 2/1(fix_headingError) -> " 13"/1
  [ic_alt] -> coord_err7/4(alt)
  Demux6/8 -> heading_err    8/1
  [ic_lon] -> coord_err8/2(dlon)
  [SINS_heading] -> heading_err1/1, heading_3/1
  crtl_Vn1/1 -> "   35"/2, "Vn_err  "/2
  [ctrl_data] -> Demux5/1
  Demux5/5 -> lon_err3/2, "   38"/2
  Pitch_1/1 -> pitch_err_FBon1/1, " 15"/1
  pitch_err 1/1 -> To Workspace17/1, "   26"/1
  "Vh_err  "/1 -> "   30"/1, Vh_err 1/1(data_in)
  [ic_lat] -> coord_err8/3(lat)
  lat_err4/1 -> coord_err7/1(dlat)
  Roll_err   1/1 -> "   46"/1, "roll_err     "/1(data_in), "   29"/1
  heading_err    1/1 -> heading_err  1/1(headingError)
  alt_err 1/1(data_out) -> To Workspace36/1, "   24"/1
  heading_err    2/1 -> heading_err     2/1(data_in)
  Demux5/4 -> lat_err3/2, "   37"/2
  "alt_err    "/1 -> "   43"/1, alt_err 1/1(data_in)
  heading_3/1 -> " 16"/1, heading_err_FBon1/1
  d_roll1/1 -> "   27"/2
  "Ve_err   "/1 -> "   33"/1, Ve_err 1/1(data_in)
  heading_err  1/1(fix_headingError) -> "   44"/1, "heading_err     "/1(data_in)
  [SINS_longitude] -> lon_err4/1
  lon_err 1/1(data_out) -> lat_err 2/2(dLon), Scope8/2, To Workspace35/1
  [SINS_Vn] -> "   35"/1, "Vn_err  "/1
  roll_err6/1 -> Pitch_err   1/1
  heading_5/1 -> "   36"/1
  roll_err 1/1 -> To Workspace18/1, "   27"/1
  [d_yaw] -> heading_err    2/1
  [SINS_longitude] -> lon_err3/1, "   38"/1
  [d_roll] -> heading_err    4/1
  "roll_err     "/1(data_out) -> "   41"/1
  bigHeadingFix2/1(fix_headingError) -> heading_6/1, heading_5/1, heading_4/1, roll_err7/1
  crtl_altitude1/1 -> "   39"/2, "alt_err    "/2
  heading_err    3/1 -> heading_err     3/1(data_in)
  d_pitch1/1 -> "   26"/2
  Demux6/1 -> To Workspace20/1
  heading_err    7/1 -> To Workspace28/1
  coord_err8/1(x) -> To Workspace23/1
  heading_err     2/1(data_out) -> To Workspace15/1
  heading_err1/1 -> bigHeadingFix2/1(headingError)
  Pitch_err   1/1 -> "   45"/1, "pitch_err    "/1(data_in), "   28"/1
  heading_err    6/1 -> To Workspace29/1
  heading_err    9/1 -> To Workspace26/1
  [SINS_latitude] -> lat_err4/1
  heading_err     1/1(data_out) -> "   47"/1
  heading_err    8/1 -> To Workspace27/1
  [ic_lon] -> heading_err    5/1
  [ic_lat] -> coord_err7/3(lat)
  seter6/1(signal) -> "roll_err     "/2(ctrl)
  lat_err3/1 -> Radians to Degrees22/1
  crtl_Vh1/1 -> "   23"/2, "Vh_err  "/2
  heading_INS  2/1(fix_headingError) -> To Workspace37/1, "   48"/1, heading_err     1/1(data_in)
  heading_err    4/1 -> heading_err     4/1(data_in)
  seter12/1(signal) -> heading_err     3/2(ctrl)
  [ctrl_data] -> Demux6/1
  seter3/1(signal) -> Vh_err 1/2(ctrl)
  lon_err4/1 -> coord_err7/2(dlon)
  seter9/1(signal) -> heading_err     1/2(ctrl)
  Demux5/8 -> Radians to Degrees29/1, pitch_err1/2
  seter10/1(signal) -> alt_err 1/2(ctrl)
  seter13/1(signal) -> heading_err     2/2(ctrl)
  [d_pitch] -> d_pitch1/1, roll_err6/2
  Demux5/7 -> bigHeadingFix1/1(heading_bad)
  "pitch_err    "/1(data_out) -> "   42"/1
  roll_err7/1 -> heading_err    1/1
  Demux5/2 -> crtl_Vn1/1
  seter8/1(signal) -> "heading_err     "/2(ctrl)
  Vn_err 1/1(data_out) -> Display29/1, To Workspace32/1, "   40"/1
  roll_1/1 -> roll_err_FBon1/1, " 14"/1
  heading_INS  1/1(fix_headingError) -> "   25"/1
  seter2/1(signal) -> Vn_err 1/2(ctrl)
  [ic_lat] -> coord_err8/1(dlat)
  Demux6/3 -> To Workspace22/1
  Radians to Degrees28/1 -> roll_err_FBon1/2, " 14"/2
  Radians to Degrees27/1 -> Display32/1, "  3"/1
  pitch_err1/1 -> pitch_err 1/1, roll_err6/1
  seter11/1(signal) -> heading_err     4/2(ctrl)
  Radians to Degrees22/1 -> "   21"/1, Display31/1
  Demux6/2 -> To Workspace21/1
  [ic_lon] -> lon_err4/2
  [SINS_altitude] -> "   39"/1, "alt_err    "/1
  [SINS_latitude] -> "   37"/1, lat_err3/1
  lon_err3/1 -> Radians to Degrees27/1
  heading_err_FBon1/1 -> heading_err_FBon 2/1(headingError)
  Demux6/6 -> coord_err8/4(alt), To Workspace25/1
  Radians to Degrees21/1 -> d_heading1/1
  Vh_err 1/1(data_out) -> To Workspace33/1, Display30/1, "   22"/1
  Demux6/9 -> heading_err    7/1
  d_heading1/1 -> "   25"/2
  coord_err7/1(x) -> Scope9/1, lat_err 1/1(data_in)
  coord_err8/2(y) -> To Workspace24/1
  [ic_lat] -> heading_err    6/1
  Demux5/6 -> crtl_altitude1/1
  Radians to Degrees31/1 -> heading_err_FBon1/2, " 16"/2
  heading_4/1 -> heading_INS  1/1(headingError)
  Demux5/1 -> crtl_Ve1/1
  "heading_err     "/1(data_out) -> "   32"/1
  Demux5/9 -> roll_err4/2, Radians to Degrees28/1
  [d_pitch] -> heading_err    3/1
  Radians to Degrees29/1 -> pitch_err_FBon1/2, " 15"/2
  heading_err     4/1(data_out) -> To Workspace19/1
  Demux6/7 -> heading_err    9/1
  seter7/1(signal) -> "pitch_err    "/2(ctrl)
  lat_err 1/1(data_out) -> lat_err 2/1(dLat), Scope8/1, To Workspace34/1
  heading_err     3/1(data_out) -> To Workspace6/1
  roll_err5/1 -> Roll_err   1/1
  roll_err4/1 -> roll_err5/1, roll_err 1/1
  "Vn_err  "/1 -> "   31"/1, Vn_err 1/1(data_in)
  Constant34/1 -> Fuck matlab8/4(errSize)
  Demux/24 -> Mux/1, Scope11/1
  [satIDvis] -> ADD error SAT/5(satID)
  ADD error SAT/1(psdRange_spuff) -> [psdRangeSat_spuf]
  [corruptSatCount] -> ADD error SAT/2(corruptSatCount)
  [errVal] -> ADD error SAT/4(errVal)
  From270/1 -> Fuck matlab10/2(psdRangeSat)
  From289/1 -> Fuck matlab10/3(satCoefs)
  From291/1 -> Fuck matlab10/1(satID)
  From298/1 -> Fuck matlab10/4(satInctrl)
  [satInctrl] -> ADD error SAT/7(satInctrl)
  [psdRange_SATvis] -> ADD error SAT/3(psdRange_SATvis)
  Fuck matlab8/1(corruptValue) -> To Workspace4/1, [errVal]
  seter1/1(signal) -> Ve_err 1/2(ctrl)
  [time_shift] -> seter1/1(time_shift)
  [time_shift] -> seter2/1(time_shift)
  [time_shift] -> seter3/1(time_shift)
  [time_shift] -> seter5/1(time_shift)
  seter5/1(signal) -> lat_err 1/2(ctrl)
  [time_shift] -> seter4/1(time_shift)
  seter4/1(signal) -> lon_err 1/2(ctrl)
  [time_shift] -> seter9/1(time_shift)
  [time_shift] -> seter8/1(time_shift)
  [time_shift] -> seter7/1(time_shift)
  [time_shift] -> seter6/1(time_shift)
  [time_shift] -> seter11/1(time_shift)
  [time_shift] -> seter12/1(time_shift)
  [time_shift] -> seter13/1(time_shift)
  [time_shift] -> seter10/1(time_shift)
  [satStartTime] -> GNNS_freq_imitetor/5(tStart)
  [satStopTime] -> GNNS_freq_imitetor/6(tEnd)
  [satStartTime] -> GNSS_integrity_control1/19(satStartTime)
  [time_shift] -> GNSS_integrity_control1/20(time_shift)
  [SINS_latitude] -> To Workspace3/1
  [SINS_longitude] -> To Workspace42/1
  [SINS_altitude] -> To Workspace43/1
  MATLAB Function3/21(satStop) -> Goto136/1
  MATLAB Function3/20(satStart) -> Goto112/1
  MATLAB Function3/23(satDeltaDown) -> Goto146/1
  MATLAB Function3/22(satDeltaUp) -> Goto145/1
  GNNS_freq_imitetor1/1(dispSatReal) -> [DispSat]
  [satStartTime] -> GNNS_freq_imitetor1/2(satStart)
  [satStopTime] -> GNNS_freq_imitetor1/3(satStop)
  [satDeltaUp] -> GNNS_freq_imitetor1/4(satDeltaUp)
  [satDeltaDown] -> GNNS_freq_imitetor1/5(satDeltaDown)
  [time_shift] -> GNNS_freq_imitetor1/6(timeStep)
  MATLAB Function3/17(Ve_off) -> Goto137/1
  MATLAB Function3/18(Vn_off) -> Goto129/1
  MATLAB Function3/19(Vh_off) -> Goto138/1
  MATLAB Function3/14(lat_off) -> Goto139/1
  MATLAB Function3/15(lon_off) -> Goto140/1
  MATLAB Function3/16(alt_off) -> Goto141/1
  Constant17/1 -> Fuck matlab3/2(criteria)
  Fuck matlab3/1(data_fix) -> Scope13/1
  Constant28/1 -> Fuck matlab4/2(criteria)
  Fuck matlab4/1(data_fix) -> Scope14/1
  GNSS_integrity_control1/4(fastLevel) -> Fuck matlab4/1(data), To Workspace41/1
  Constant29/1 -> Fuck matlab11/2(criteria)
  Fuck matlab11/1(data_fix) -> Scope10/1
  GNSS_integrity_control1/3(fastCritLevel) -> Fuck matlab11/1(data), To Workspace39/1
  MATLAB Function4/19(Vh_off) -> [offSet_Vh]
  MATLAB Function4/23(satDeltaDown) -> [satDeltaDown]
  MATLAB Function4/20(satStart) -> [satStartTime]
  MATLAB Function4/18(Vn_off) -> [offSet_Vn]
  MATLAB Function4/16(alt_off) -> [offSet_alt]
  MATLAB Function4/15(lon_off) -> [offSet_lon]
  MATLAB Function4/21(satStop) -> [satStopTime]
  MATLAB Function4/14(lat_off) -> [offSet_lat]
  MATLAB Function4/17(Ve_off) -> [offSet_Ve]
  MATLAB Function4/3(heading) -> [ic_heading]
  MATLAB Function4/8(Ve) -> [ic_Ve]
  MATLAB Function4/1(GRS) -> [GRS_data]
  MATLAB Function4/9(Vn) -> [ic_Vn]
  MATLAB Function4/6(lat) -> [ic_lat]
  MATLAB Function4/22(satDeltaUp) -> [satDeltaUp]
  MATLAB Function4/7(lon) -> [ic_lon]
  MATLAB Function4/5(roll) -> [ic_roll]
  MATLAB Function4/4(pitch) -> [ic_pitch]
  MATLAB Function4/11(Vh) -> [ic_Vh]
  MATLAB Function4/2(ACC) -> [ACC_data]
  MATLAB Function4/12(time_shft) -> [time_shift]
  MATLAB Function4/13(cntrl_data) -> [ctrl_data]
  MATLAB Function4/10(H) -> [ic_alt]
  [ctrl_pos] -> Terminator9/1
  [ctrl_vel] -> Terminator10/1
  [ctrl_ang] -> Terminator11/1
  [ctrl_alt] -> Terminator12/1
  Demux6/5 -> Terminator18/1
  Demux6/4 -> Terminator19/1
  Model2/10 -> Terminator21/1
  Model2/11 -> Terminator22/1
  Model2/12 -> Terminator23/1
  Model2/13 -> Terminator24/1
  Constant30/1 -> Scope87/5
  MATLAB Function4/26(corruptPSDError) -> [corruptPSDError]
  MATLAB Function4/24(corruptSatCount) -> [corruptSatCount]
  MATLAB Function4/25(corruptTimeStart) -> [corruptTimeStart]
  MATLAB Function4/27(corruptErrorType) -> [corruptErrorType]
  [corruptErrorType] -> Fuck matlab8/7(corruptErrorType)
  [corruptPSDError] -> Fuck matlab8/6(corruptPSDError)
  [corruptTimeStart] -> Fuck matlab8/5(corruptTimeStart)
  [time_shift] -> Fuck matlab8/8(dt)
  Constant35/1 -> psdRange_Sat/14
  Constant36/1 -> psdRange_Sat1/14
  [offSet_lat] -> psdRange_Sat/12
  [offSet_lon] -> psdRange_Sat/13
  MATLAB Function4/28(K_fastCircle_psd) -> [K_fast_psd]
  MATLAB Function4/29(K_fastCircle_psd_dot) -> [K_fast_psd_dot]
  [K_fast_psd] -> Mux3/1
  [K_fast_psd_dot] -> Mux3/2
  [K_slowSensivity] -> Mux3/3
  [K_slowWindow] -> Mux3/4
  MATLAB Function4/30(K_slowWindow) -> [K_slowWindow]
  MATLAB Function4/31(K_slowSensivity) -> [K_slowSensivity]
  Mux3/1 -> GNSS_integrity_control1/21(sensitivity)
  Constant16/1 -> Terminator20/1
  Fuck matlab2/1(data_fix) -> Scope1/1
  GNSS_integrity_control1/6(z_level) -> Fuck matlab2/1(data), To Workspace2/1
  Constant6/1 -> Fuck matlab2/2(criteria)
  Constant7/1 -> Fuck matlab1/2(criteria)
  Fuck matlab1/1(data_fix) -> Scope2/1
  [posObj] -> DOPS/5(posObj)
  ADD error SAT/2(LQE_Z_spuff) -> DOPS/2(satInfo), GNNS_freq_imitetor/2(satInfo_AV)
  [satCoefs] -> ADD error SAT/6(satCoefs)
  bigHeadingFix1/1(heading_norm) -> heading_err1/2, Radians to Degrees31/1
  [SINS_longitude] -> psdRange_Sat1/13
  [SINS_latitude] -> psdRange_Sat1/12
  GSK->DGSK/1(pos) -> [posObj]
  [posObj] -> psdRange_Sat/4
  GNSS_integrity_control1/7(z_crout) -> Fuck matlab1/1(data), To Workspace44/1
  Fuck matlab10/1(psdRange_fix) -> Terminator26/1
  [satCountPreset] -> Fuck matlab11/3(satCountPreset)
  [satCountPreset] -> Fuck matlab4/3(satCountPreset)
  [satCountPreset] -> Fuck matlab3/3(satCountPreset)
  [satCountPreset] -> Fuck matlab2/3(satCountPreset)
  [satCountPreset] -> Fuck matlab1/3(satCountPreset)
  DOPS/5(DOP) -> Terminator17/1
  [offSet_Vh] -> GSK->DGSK/6(Vh)
  [offSet_Vn] -> GSK->DGSK/5(Vn)
  [offSet_Ve] -> GSK->DGSK/4(Ve)
  [offSet_alt] -> GSK->DGSK/3(alt)
  [offSet_lon] -> GSK->DGSK/2(lon)
  [offSet_lat] -> GSK->DGSK/1(lat)
  [SINS_Vn] -> GSK->DGSK1/5(Vn)
  [SINS_Vh] -> GSK->DGSK1/6(Vh)
  [SINS_Ve] -> GSK->DGSK1/4(Ve)
  [SINS_altitude] -> GSK->DGSK1/3(alt)
  [SINS_longitude] -> GSK->DGSK1/2(lon)
  [SINS_latitude] -> GSK->DGSK1/1(lat)
  [dPsdRange] -> altimetrImitator1/1(psdRangeNoise)
  [lqe_P] -> Terminator8/1
  [dKgrs] -> Terminator13/1
  [dKacc] -> Terminator14/1
  [dgrs] -> Terminator15/1
  [dacc] -> Terminator16/1
  [sigmPrdRange] -> Terminator27/1
  Constant15/1 -> Model2/36
  Memory1/1 -> [ctrlSatCoefs]
  Model2/22 -> Memory1/1
  [ctrlSatCoefs] -> ADD error SAT/8(ctrlSatCoefs)
  lat_err 2/1(crdErr) -> To Workspace46/1
  [offSet_lat] -> Scope3/2
  [offSet_lon] -> Scope3/1

== matlab function base_model_lqeH/Fuck matlab11 ==
  data: data_fix output size=8; data input; criteria input; satCountPreset input
function data_fix =  forCtrl(data, criteria, satCountPreset)
    
    data_fix = zeros(8,1);
    for ii = 1:8
        if data(ii) > criteria
            data(ii) = nan;
        end
    end
    data_fix = data;    
end

== matlab function base_model_lqeH/INS mesurment model ==
  data: grs_ideal input; grs_data output; acc_ideal input; acc_data output; dacc output; dgrs output; dK_acc output; dK_grs output; n1 input; n2 input; n3 input; n4 input
function [grs_data, acc_data, dacc, dgrs, dK_acc, dK_grs]= INS_mesure_err (grs_ideal, acc_ideal, n1,n2,n3,n4)


    %парметры модели погрешности измерений ДУС и акселерометров
    dacc      = 0.004;
    dgrs      = 4.5*1e-6;
    grs_noise = deg2rad(0.15*1e-5)/60;
    acc_noise = 1e-5;
    dK_acc    = 3*1e-4;
    dK_grs    = 5*1e-4;

    d_acc = ones(size(acc_ideal)).*dacc;
    d_grs = ones(size(grs_ideal)).*dgrs;

    acc_data = zeros(3,1);
    grs_data = zeros(3,1);

    acc_data = acc_ideal + d_acc + dK_acc.*acc_ideal + acc_noise.*randn(size(acc_ideal))/5;
    grs_data = grs_ideal + d_grs + dK_grs.*grs_ideal + grs_noise.*randn(size(grs_ideal))/5;

end

== matlab function base_model_lqeH/lqe_coord_cor2 ==
  data: heading input; pitch input; roll input; heading_0 output; pitch_0 output; roll_0 output; lat input; lon input; alt input; Ve input; Vn input; Vh input; lat_0 output; lon_0 output; alt_0 output; Ve_0 output; Vn_0 output; Vh_0 output
function [heading_0,pitch_0,roll_0,lat_0,lon_0,alt_0,Ve_0,Vn_0,Vh_0] =INS_mesure_err(heading,pitch,roll,lat, lon,alt,Ve,Vn, Vh)
    
    lat_0     = lat     + deg2rad(10/6378136);
    lon_0     = lon     + deg2rad(10/(6378136)*cos(lat));
    alt_0     = alt     + 5;
    Ve_0      = Ve      + 0.77;%0.05;
    Vn_0      = Vn      + 0.77;%0.05;
    Vh_0      = Vh      + 0.06;%0.05;
    heading_0 = heading + deg2rad(0.25);%deg2rad(0.25);
    pitch_0   = pitch   + deg2rad(0.03);%deg2rad(0.03);
    roll_0    = roll    + deg2rad(0.03);%deg2rad(0.03);
    

end

== matlab function base_model_lqeH/lat_err 2 ==
  data: crdErr output size=1; dLat input; dLon input
function crdErr  = slowData(dLat, dLon)
 
    crdErr = sqrt(dLat.^2 + dLon.^2);
    
end

== matlab function base_model_lqeH/StaPosition ==
  data: satCounter output; time_shift input; satPosVel output size=6,32; satHealth output size=32
function [satCounter, satPosVel, satHealth]= ALM_read(time_shift)

    persistent data time U

    if isempty(data)
        data  = load('Almanac_parsed.mat');    %lol thnx to Savkin
        time = 0;
        U = deg2rad((360/24)/3600);
        a  = 0;%zeros(length(data.al_gp_e(:,1)),1);
        et = zeros(length(data.al_gp_e(:,1)),1);
        mt = zeros(length(data.al_gp_e(:,1)),1);
    end


    satCounter      = length(data.al_gp_e(:,1));
    satPosVel       = zeros(6,32); % [pos_X,pos_Y,pos_Z,vel_X,vel_Y,vel_Z]
    satHealth       = zeros(32,1);
    
    A = inv([cos(U * time), -sin(U * time), 0;
             sin(U * time),  cos(U * time), 0;
             0,          0,                 1]);
    
    time = time + time_shift;
    dt = (time);
    
    for ii = 1:satCounter
        a      = data.al_gp_sqrt_a(ii).^2;
        mt(ii) = data.al_gp_m0(ii) + dt .* sqrt(data.al_gp_mu ./ a.^3);
        et(ii) = mt(ii);

%         for jj = 0:(data.al_gp_resolution / 100)-1
            et(ii) = et(ii) - (et(ii) - data.al_gp_e(ii) .* sin(et(ii)) - mt(ii)) ...
                /  (1 - data.al_gp_e(ii) .* (cos(et(ii))));
%         end

        vt = 2 .* atan2(sqrt(1 + data.al_gp_e(ii))*sin(et(ii)./ 2), sqrt(1 - data.al_gp_e(ii)) * cos(et(ii) ./ 2));
        rt = a .* (1 - data.al_gp_e(ii) .* cos(et(ii)));

        ot_x = rt .* cos(vt);
        ot_y = rt .* sin(vt);

        d_ot_x = (sqrt(data.al_gp_mu .* a) ./ rt) .* (-sin(et(ii)));
        d_ot_y = (sqrt(data.al_gp_mu .* a) ./ rt) .* (sqrt(1 - data.al_gp_e(ii) .^2 ) * cos(et(ii)));


        pos = [(ot_x.*(cos(data.al_gp_w(ii)).*cos(data.al_gp_lan(ii)) - sin(data.al_gp_w(ii)).*cos(data.al_gp_i(ii)).*sin(data.al_gp_lan(ii))) - ot_y.*(sin(data.al_gp_w(ii)).*cos(data.al_gp_lan(ii)) + cos(data.al_gp_w(ii)).*cos(data.al_gp_i(ii)).*sin(data.al_gp_lan(ii)))); 
               (ot_x.*(cos(data.al_gp_w(ii)).*sin(data.al_gp_lan(ii)) + sin(data.al_gp_w(ii)).*cos(data.al_gp_i(ii)).*cos(data.al_gp_lan(ii))) + ot_y.*(cos(data.al_gp_w(ii)).*cos(data.al_gp_i(ii)).*cos(data.al_gp_lan(ii)) - sin(data.al_gp_w(ii)).*sin(data.al_gp_lan(ii)))); 
               (ot_x.*(sin(data.al_gp_w(ii)).*sin(data.al_gp_i(ii))) + ot_y.*(cos(data.al_gp_w(ii)).*sin(data.al_gp_i(ii))))];

        vel = [(d_ot_x.*(cos(data.al_gp_w(ii)).*cos(data.al_gp_lan(ii)) - sin(data.al_gp_w(ii)).*cos(data.al_gp_i(ii)).*sin(data.al_gp_lan(ii))) - d_ot_y.*(sin(data.al_gp_w(ii)).*cos(data.al_gp_lan(ii)) + cos(data.al_gp_w(ii)).*cos(data.al_gp_i(ii)).*sin(data.al_gp_lan(ii)))); 
               (d_ot_x.*(cos(data.al_gp_w(ii)).*sin(data.al_gp_lan(ii)) + sin(data.al_gp_w(ii)).*cos(data.al_gp_i(ii)).*cos(data.al_gp_lan(ii))) + d_ot_y.*(cos(data.al_gp_w(ii)).*cos(data.al_gp_i(ii)).*cos(data.al_gp_lan(ii)) - sin(data.al_gp_w(ii)).*sin(data.al_gp_lan(ii)))); 
               (d_ot_x.*(sin(data.al_gp_w(ii)).*sin(data.al_gp_i(ii)))  + d_ot_y.*(cos(data.al_gp_w(ii)).*sin(data.al_gp_i(ii))))];

           
           
        pos_x_dgsk = A(1,1) * pos(1) + A(1,2) * pos(2) + A(1,3) * pos(3);
        pos_y_dgsk = A(2,1) * pos(1) + A(2,2) * pos(2) + A(2,3) * pos(3);
        pos_z_dgsk = A(3,1) * pos(1) + A(3,2) * pos(2) + A(3,3) * pos(3);
           
        satPosVel(:,ii) = [pos_x_dgsk,pos_y_dgsk,pos_z_dgsk,vel(1),vel(2),vel(3)];   
        satHealth(ii)   = data.al_gp_health(ii);
         
    end
end

== matlab function base_model_lqeH/GSK->DGSK1 ==
  data: pos output size=3; lat input; lon input; alt input; Ve input; Vn input; Vh input; vel output
function [pos, vel]= getDGSK(lat, lon, alt, Ve, Vn, Vh)

    pos = zeros(3,1);
    vel = zeros(3,1);
    
    b  = 6356751.3618;
    a  = 6378136;
    e2 = (a^2 - b^2)/a^2;%double(0.0066943662); 

    N = (a) ./ sqrt(1-e2*(sin(lat).^2));
    %N = (a^2) ./ sqrt((a^2)*(cos(lat))^2 + (b^2)*(sin(lat)^2));


    X = (N + alt)*cos(lat)*cos(lon);
    Y = (N + alt)*cos(lat)*sin(lon);
    Z = (((b^2)/(a^2))*N + alt)*sin(lat);

    velRec = zeros(3,3);
    velRec = [-sin(lon), -cos(lon) * sin(lat), cos(lon) * cos(lat); 
               cos(lon), -sin(lon) * sin(lat), sin(lon) * cos(lat);
                      0,             cos(lat), sin(lat)];
    
    
   
    vel = velRec*[Ve; Vn; Vh];
    
    pos(1) = X;
    pos(2) = Y;
    pos(3) = Z;
end

== matlab function base_model_lqeH/GSK->DGSK ==
  data: pos output size=3; lat input; lon input; alt input; Ve input; Vn input; Vh input; vel output
function [pos, vel]= getDGSK(lat, lon, alt, Ve, Vn, Vh)

    pos = zeros(3,1);
    vel = zeros(3,1);
    
    b  = 6356751.3618;
    a  = 6378136;
    e2 = (a^2 - b^2)/a^2;%double(0.0066943662); 

    N = (a) ./ sqrt(1-e2*(sin(lat).^2));
    %N = (a^2) ./ sqrt((a^2)*(cos(lat))^2 + (b^2)*(sin(lat)^2));


    X = (N + alt)*cos(lat)*cos(lon);
    Y = (N + alt)*cos(lat)*sin(lon);
    Z = (((b^2)/(a^2))*N + alt)*sin(lat);

    velRec = zeros(3,3);
    velRec = [-sin(lon), -cos(lon) * sin(lat), cos(lon) * cos(lat); 
               cos(lon), -sin(lon) * sin(lat), sin(lon) * cos(lat);
                      0,             cos(lat), sin(lat)           ];
    
    
   
    vel = velRec*[Ve; Vn; Vh];
    
    pos(1) = X;
    pos(2) = Y;
    pos(3) = Z;
end
